simulink model "simulink_discrete"  (R2021a)
settings: Solver=ode45  StartTime=0.0  StopTime=0.7  RelTol=1e-3  EnableMultiTasking=on
undefined symbols (not defined in the file): a1, a2, b0, b1, b2, Ts2
libraries: cstblocks x4
settings Model: Creator=Koldo  LastModifiedBy=EIB
settings SolverCC: AlgebraicLoopSolver=TrustRegion
settings DataIOCC: LimitDataPoints=on  SaveFormat=Array  SignalLoggingSaveFormat=ModelDataLogs  ReturnWorkspaceOutputs=off
settings OptimizationCC: ExpressionDepthLimit=2147483647  LifeSpan=inf
settings DebuggingCC: UnderspecifiedInitializationDetection=Classic  MergeDetectMultiDrivingBlocksExec=none  SolverPrmCheckMsg=warning  FcnCallInpInsideContextMsg=warning  StateNameClashWarn=warning  SFUnexpectedBacktrackingDiag=warning  SFNoUnconditionalDefaultTransitionDiag=warning  SFExecutionAtInitializationDiag=none  SFMachineParentedDataDiag=warning  ArithmeticOperatorsInVariantConditions=warning
settings HardwareCC: ProdBitPerPointer=32  ProdBitPerSizeT=32  ProdBitPerPtrDiffT=32  ProdLargestAtomicFloat=None  ProdIntDivRoundTo=Undefined  ProdEndianess=Unspecified  ProdWordSize=32  ProdHWDeviceType=32-bit Generic
settings ModelReferenceCC: PropagateSignalLabelsOutOfModel=off
settings SFSimCC: SimUseLocalCustomCode=off  CustomCodeUndefinedFunction=UseInterfaceOnly
settings RTWCC: RTWUseLocalCustomCode=off
settings CodeAppCC: StateflowObjectComments=on
settings GRTTargetCC: TargetLangStandard=C89/C90 (ANSI)  CombineOutputUpdateFcns=off  GRTInterface=on
settings ConfigComp: CovMetricSettings=dw  CovSaveCumulativeToWorkspaceVar=on  CovSaveSingleToWorkspaceVar=on  CovExternalEMLEnable=off

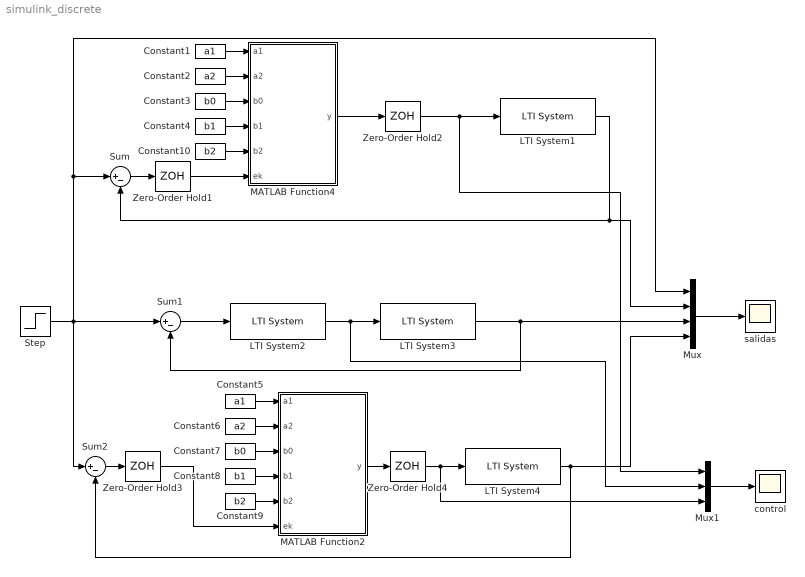
== system simulink_discrete ==
  Constant1 : Constant  Value=a1
  Constant10 : Constant  Value=b2
  Constant2 : Constant  Value=a2
  Constant3 : Constant  Value=b0
  Constant4 : Constant  Value=b1
  Constant5 : Constant  Value=a1
  Constant6 : Constant  Value=a2
  Constant7 : Constant  Value=b0
  Constant8 : Constant  Value=b1
  Constant9 : Constant  Value=b2
  LTI System1 : cstblocks/LTI System  sys=G_s  IC=[]
  LTI System2 : cstblocks/LTI System  sys=C_s  IC=[]
  LTI System3 : cstblocks/LTI System  sys=G_s  IC=[]
  LTI System4 : cstblocks/LTI System  sys=G_s  IC=[]
  MATLAB Function2 : MATLAB Function  TreatAsAtomicUnit=on
  MATLAB Function4 : MATLAB Function  TreatAsAtomicUnit=on
  Mux : Mux
  Mux1 : Mux  Inputs=3
  Step : Step  Time=0  After=pi  SampleTime=0
  Sum : Sum  Inputs=|+-
  Sum1 : Sum  Inputs=|+-
  Sum2 : Sum  Inputs=|+-
  Zero-Order Hold{1..4} (4 alike) : ZeroOrderHold  SampleTime=Ts2
  control : Scope
  salidas : Scope
  wires:
  Sum/1 -> Zero-Order Hold1/1
  LTI System1/1 -> Mux/2, Sum/2
  Zero-Order Hold2/1 -> LTI System1/1, Mux1/1
  Step/1 -> Sum2/1, Sum1/1, Sum/1, Mux/1
  Sum1/1 -> LTI System2/1
  LTI System3/1 -> Sum1/2, Mux/3
  LTI System2/1 -> LTI System3/1, Mux1/2
  Mux/1 -> salidas/1
  Sum2/1 -> Zero-Order Hold3/1
  LTI System4/1 -> Mux/4, Sum2/2
  Zero-Order Hold3/1 -> MATLAB Function2/6(ek)
  Zero-Order Hold4/1 -> LTI System4/1, Mux1/3
  Mux1/1 -> control/1
  Constant8/1 -> MATLAB Function2/4(b1)
  Constant5/1 -> MATLAB Function2/1(a1)
  Constant9/1 -> MATLAB Function2/5(b2)
  Constant7/1 -> MATLAB Function2/3(b0)
  Constant6/1 -> MATLAB Function2/2(a2)
  MATLAB Function2/1(y) -> Zero-Order Hold4/1
  Constant4/1 -> MATLAB Function4/4(b1)
  Constant10/1 -> MATLAB Function4/5(b2)
  Constant2/1 -> MATLAB Function4/2(a2)
  Constant1/1 -> MATLAB Function4/1(a1)
  Constant3/1 -> MATLAB Function4/3(b0)
  Zero-Order Hold1/1 -> MATLAB Function4/6(ek)
  MATLAB Function4/1(y) -> Zero-Order Hold2/1

== matlab function simulink_discrete/MATLAB Function4 ==
  data: a1 input; a2 input; b0 input; b1 input; b2 input; y output; ek input
function y = fcn(a1,a2,b0,b1,b2,ek)

    

    % Registros 1D
    persistent pk1 pk2
    % Forma canónica (2 registros). Sensible a la cuantificación numérica.
    % uk = b0(ek-a1*pk1-a2*pk2) + b1*pk1 + b2*pk2;
    % Inicializamos los registros (reset)
    if isempty (pk1)
        pk1=0;
    end
    if isempty (pk2)
        pk2=0;
    end
    
    %Realimentación
    %ek = setpoints - yk;
    
    %Cálculo de la señal de control
    apk1 = a1*pk1;
    apk2 = a2*pk2;
    pk = ek - apk1 - apk2;
    
    bpk = b0*pk;
    bpk1 = b1*pk1;
    bpk2 = b2*pk2;
    uk = bpk + bpk1 + bpk2;
    
    %Actualizamos los registros
    pk2=pk1;
    pk1=pk;
    u=uk;
y = u;

== matlab function simulink_discrete/MATLAB Function2 ==
  data: a1 input; a2 input; b0 input; b1 input; b2 input; y output; ek input
function y = fcn(a1,a2,b0,b1,b2,ek)
    

    persistent ek1 ek2 uk1 uk2
    % No canónica: cuatro registros
    % u(k) = b0*e(k)+b1*e(k-1)+b2*e(k-2)-a1*u(k-1)-a2*u(k-2)
    if isempty (uk1)
        uk1=0;
     end
     if isempty (uk2)
        uk2=0;
    end
    if isempty (ek1)
        ek1=0;
    end
    if isempty (ek2)
        ek2=0;
    end

    %ek= setpoints-yk;
    uk = b0*ek+b1*ek1+b2*ek2-a1*uk1-a2*uk2;
    uk2=uk1;
    uk1=uk;
    ek2=ek1;
    ek1=ek;
    u =uk;
y = u;
